simulink model "simulink_mecha"  (R2016b)
settings: Solver=VariableStepAuto  StartTime=0.0  StopTime=50  RelTol=1e-3
libraries: aerolibutil x1, simulink x1
settings Model: Creator=Utente  LastModifiedBy=Utente

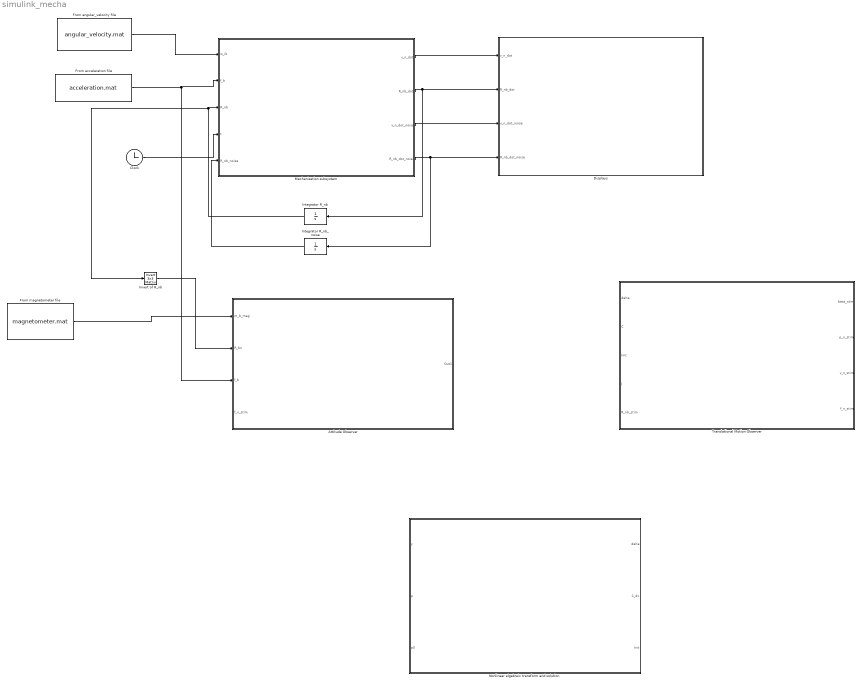
== system simulink_mecha ==
  Attitude Observer : Subsystem
  Clock : Clock
  Displays : Subsystem
  From acceleration file : FromFile  FileName=acceleration.mat  SampleTime=0
  From angular_velocity file : FromFile  FileName=angular_velocity.mat  SampleTime=0
  From magnetometer file : FromFile  FileName=magnetometer.mat  SampleTime=0  InterpolationWithinTimeRange=Zero order hold
  Integrator R_nb : Integrator
  Integrator R_nb_noise : Integrator
  Invert of R_nb : aerolibutil/Invert  3x3 Matrix
  Mechanisation subsystem : Subsystem
  Nonlinear algebraic transform and solution : Subsystem
  Translational Motion Observer : Subsystem
  wires:
  From angular_velocity file/1 -> Mechanisation subsystem/1(w_ib)
  From acceleration file/1 -> Mechanisation subsystem/2(f_b), Attitude Observer/3(f_b)
  Clock/1 -> Mechanisation subsystem/4(t)
  Mechanisation subsystem/2(R_nb_dot) -> Integrator R_nb/1, Displays/2(R_nb_dot)
  Integrator R_nb/1 -> Invert of R_nb/1, Mechanisation subsystem/3(R_nb)
  Mechanisation subsystem/1(v_n_dot) -> Displays/1(v_n_dot)
  Mechanisation subsystem/3(v_n_dot_noise) -> Displays/3(v_n_dot_noise)
  Mechanisation subsystem/4(R_nb_dot_noise) -> Integrator R_nb_noise/1, Displays/4(R_nb_dot_noise)
  Integrator R_nb_noise/1 -> Mechanisation subsystem/5(R_nb_noise)
  Invert of R_nb/1 -> Attitude Observer/2(R_bn)
  From magnetometer file/1 -> Attitude Observer/1(m_b_mag)

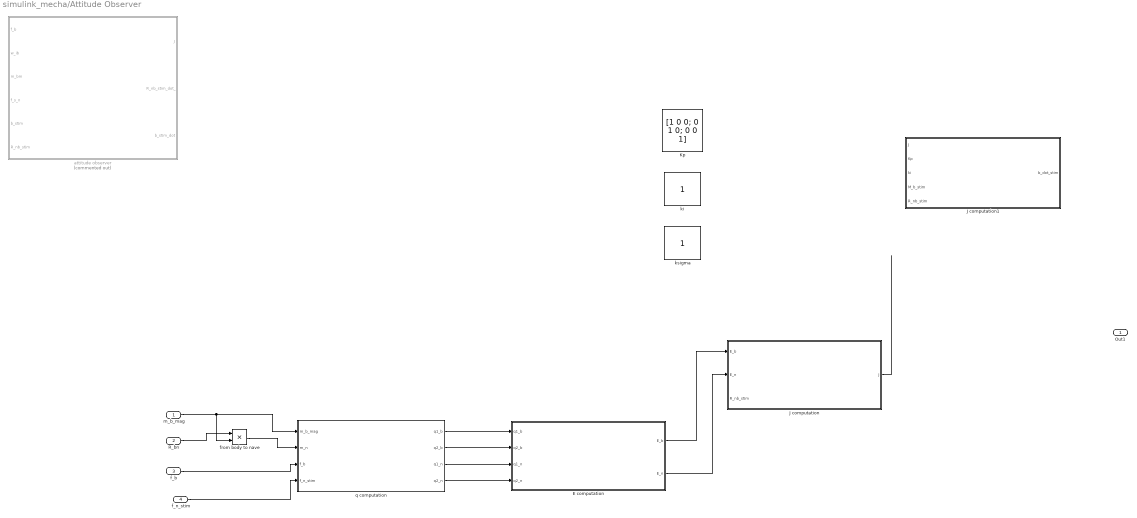
== system simulink_mecha/Attitude Observer ==
  m_b_mag : Inport
  R_bn : Inport  Port=2
  f_b : Inport  Port=3
  f_n_stim : Inport  Port=4
  E computation : MATLAB Function  TreatAsAtomicUnit=on
  J computation : MATLAB Function  TreatAsAtomicUnit=on
  J computation1 : MATLAB Function  TreatAsAtomicUnit=on
  Kp : Constant  Value=[1 0 0; 0 1 0; 0 0 1]
  attitude observer : MATLAB Function  Commented=on  TreatAsAtomicUnit=on
  from body to nave : Product
  ki : Constant
  ksigma : Constant
  q computation : MATLAB Function  TreatAsAtomicUnit=on
  Out1 : Outport
  wires:
  m_b_mag/1 -> from body to nave/2, q computation/1(m_b_mag)
  R_bn/1 -> from body to nave/1
  f_b/1 -> q computation/3(f_b)
  f_n_stim/1 -> q computation/4(f_n_stim)
  from body to nave/1 -> q computation/2(m_n)
  q computation/1(q1_b) -> E computation/1(q1_b)
  q computation/2(q2_b) -> E computation/2(q2_b)
  q computation/3(q1_n) -> E computation/3(q1_n)
  q computation/4(q2_n) -> E computation/4(q2_n)
  E computation/1(E_b) -> J computation/1(E_b)
  E computation/2(E_n) -> J computation/2(E_n)
  ? -> J computation/3(R_nb_stim)
  J computation/1(J) -> ?

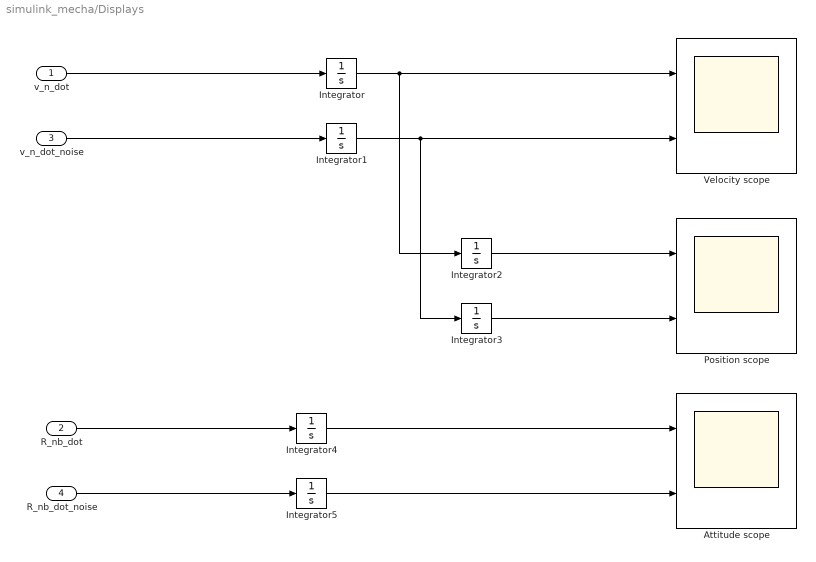
== system simulink_mecha/Displays ==
  v_n_dot : Inport
  R_nb_dot : Inport  Port=2
  v_n_dot_noise : Inport  Port=3
  R_nb_dot_noise : Inport  Port=4
  Attitude scope : Scope  NumInputPorts=2
  Integrator{,1..5} (6 alike) : Integrator
  Position scope : Scope  NumInputPorts=2
  Velocity scope : Scope  NumInputPorts=2
  wires:
  v_n_dot/1 -> Integrator/1
  v_n_dot_noise/1 -> Integrator1/1
  Integrator/1 -> Integrator2/1, Velocity scope/1
  Integrator1/1 -> Integrator3/1, Velocity scope/2
  Integrator2/1 -> Position scope/1
  Integrator3/1 -> Position scope/2
  R_nb_dot/1 -> Integrator4/1
  R_nb_dot_noise/1 -> Integrator5/1
  Integrator4/1 -> Attitude scope/1
  Integrator5/1 -> Attitude scope/2

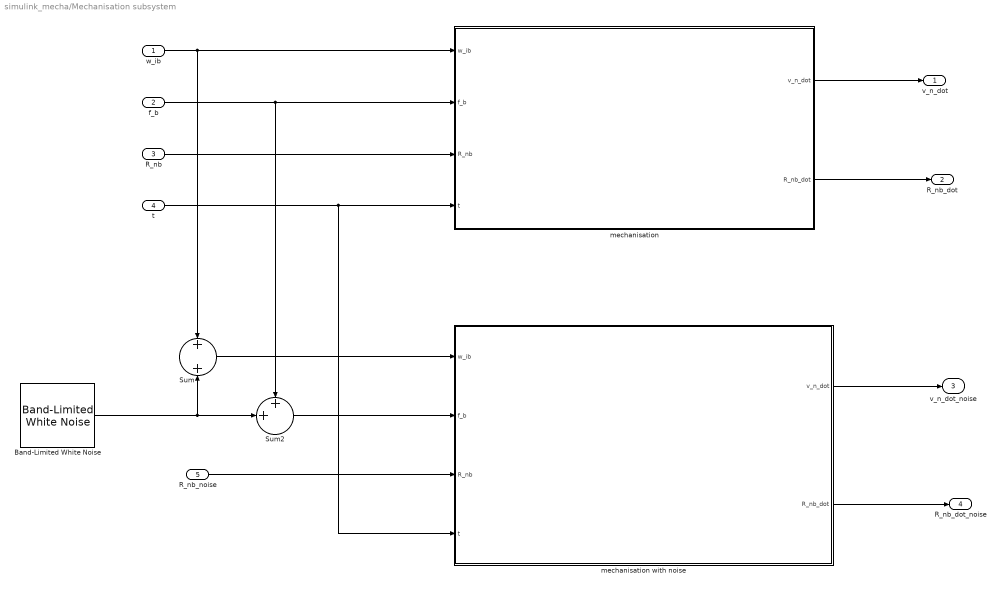
== system simulink_mecha/Mechanisation subsystem ==
  w_ib : Inport
  f_b : Inport  Port=2
  R_nb : Inport  Port=3
  t : Inport  Port=4
  R_nb_noise : Inport  Port=5
  Band-Limited White Noise : simulink/Sources/Band-Limited White Noise  Cov=[100 100 100]'  Ts=0.1  seed=[23341]  VectorParams1D=off
  Sum : Sum  Inputs=+|+
  Sum2 : Sum  Inputs=++|
  mechanisation : MATLAB Function  TreatAsAtomicUnit=on
  mechanisation with noise : MATLAB Function  TreatAsAtomicUnit=on
  v_n_dot : Outport
  R_nb_dot : Outport  Port=2
  v_n_dot_noise : Outport  Port=3
  R_nb_dot_noise : Outport  Port=4
  wires:
  w_ib/1 -> mechanisation/1(w_ib), Sum/1
  t/1 -> mechanisation with noise/4(t), mechanisation/4(t)
  R_nb/1 -> mechanisation/3(R_nb)
  f_b/1 -> Sum2/1, mechanisation/2(f_b)
  mechanisation/1(v_n_dot) -> v_n_dot/1
  mechanisation/2(R_nb_dot) -> R_nb_dot/1
  Band-Limited White Noise/1 -> Sum/2, Sum2/2
  Sum/1 -> mechanisation with noise/1(w_ib)
  Sum2/1 -> mechanisation with noise/2(f_b)
  mechanisation with noise/1(v_n_dot) -> v_n_dot_noise/1
  mechanisation with noise/2(R_nb_dot) -> R_nb_dot_noise/1
  R_nb_noise/1 -> mechanisation with noise/3(R_nb)

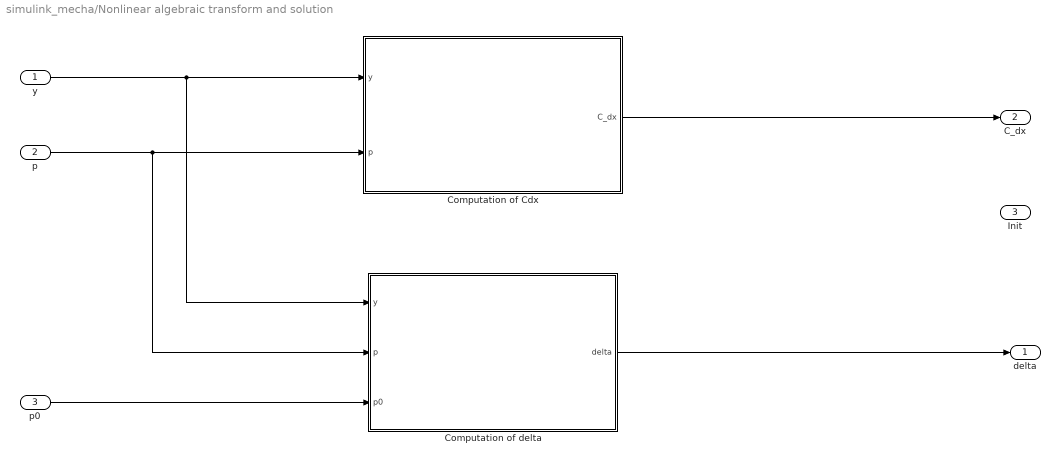
== system simulink_mecha/Nonlinear algebraic transform and solution ==
  y : Inport
  p : Inport  Port=2
  p0 : Inport  Port=3
  Computation of Cdx : MATLAB Function  TreatAsAtomicUnit=on
  Computation of delta : MATLAB Function  TreatAsAtomicUnit=on
  delta : Outport
  C_dx : Outport  Port=2
  Init : Outport  Port=3
  wires:
  y/1 -> Computation of delta/1(y), Computation of Cdx/1(y)
  p/1 -> Computation of delta/2(p), Computation of Cdx/2(p)
  p0/1 -> Computation of delta/3(p0)
  Computation of Cdx/1(C_dx) -> C_dx/1
  Computation of delta/1(delta) -> delta/1

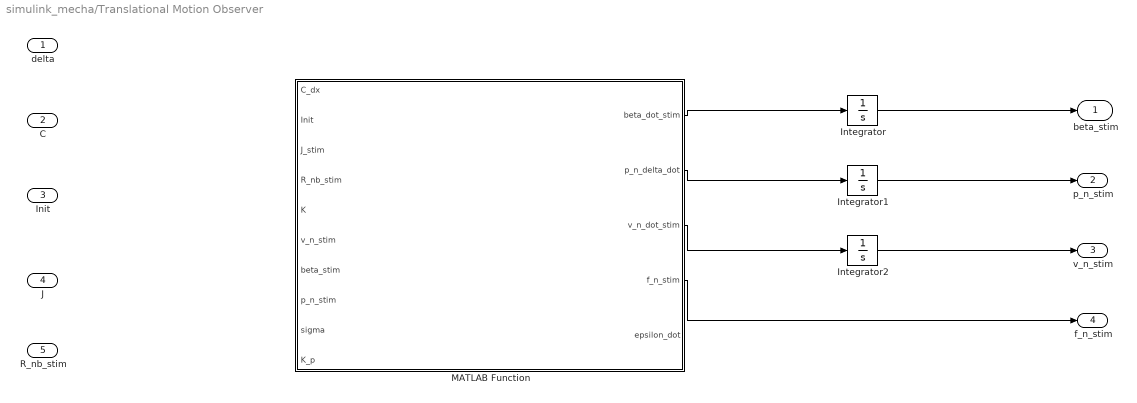
== system simulink_mecha/Translational Motion Observer ==
  delta : Inport
  C : Inport  Port=2
  Init : Inport  Port=3
  J : Inport  Port=4
  R_nb_stim : Inport  Port=5
  Integrator : Integrator
  Integrator1 : Integrator
  Integrator2 : Integrator
  MATLAB Function : MATLAB Function  TreatAsAtomicUnit=on
  beta_stim : Outport
  p_n_stim : Outport  Port=2
  v_n_stim : Outport  Port=3
  f_n_stim : Outport  Port=4
  wires:
  MATLAB Function/4(f_n_stim) -> f_n_stim/1
  MATLAB Function/3(v_n_dot_stim) -> Integrator2/1
  Integrator2/1 -> v_n_stim/1
  MATLAB Function/2(p_n_delta_dot) -> Integrator1/1
  Integrator1/1 -> p_n_stim/1
  Integrator/1 -> beta_stim/1
  MATLAB Function/1(beta_dot_stim) -> Integrator/1

== matlab function simulink_mecha/Attitude Observer/E computation ==
  data: q1_b input; E_b output; q2_b input; q1_n input; q2_n input; E_n output
function [E_b, E_n]= Efunc(q1_b, q2_b, q1_n, q2_n)



E_b = (q1_b, skew(q1_b)*q2_b, (skew(q1_b)*skew(q1_b))*q2_b);
E_n = (q1_n, skew(q1_n)*q2_n, (skew(q1_n)*skew(q1_n))*q2_n);

== matlab function simulink_mecha/Attitude Observer/q computation ==
  data: m_b_mag input; q1_b output; m_n input; f_b input; f_n_stim input; q2_b output; q1_n output; q2_n output
function [q1_b, q2_b, q1_n, q2_n] = qfunc(m_b_mag, m_n, f_b, f_n_stim)

g_n = [0 0 1]';

q1_b = m_b_mag/norm(m_b_mag,2);
q2_b = f_b/norm(g_n,2);

q1_n = m_n/norm(m_n,2);
q2_n = f_n_stim/norm(g_n,2);

== matlab function simulink_mecha/Attitude Observer/attitude observer ==
  data: f_b input; J output; w_ib input; m_bm input; f_s_n input; b_stim input; R_nb_stim input; R_nb_stim_dot_ output; b_stim_dot output
function [J, R_nb_stim_dot_, b_stim_dot] = fcn(f_b, w_ib, m_bm, f_s_n, b_stim, R_nb_stim)

g_n = [0 0 1];

Skew = zeros(3,3);
Skew(1,2) = -(w_ib(3) - b_stim(3));
Skew(2,1) = (w_ib(3) - b_stim(3));
Skew(1,3) = (w_ib(2) - b_stim(2));
Skew(3,1) = -(w_ib(2) - b_stim(2));
Skew(2,3) = -(w_ib(1) - b_stim(1));
Skew(3,2) = (w_ib(1) - b_stim(1));

Kp = eye(3); % gain matrix
sigma = 1; % sigma >= 1

J_func = eye(3);
R_nb_stim_dot = R_nb_stm * Skew + sigma * Kp * J_func;

% b_stim_dot = Proj

q1_b = m_bmag/norm(m_bmag,2);
q2_b = f_b/norm(g_n,2);

q1_n = m_n/norm(m_n,2);
q2_n = f_s_n/norm(g_n,2);



E_b = (q1_b, Skew(q1_b)*q2_b, (S(q1_b)*S(q1_b))*q2_b);
E_n = (q1_n, Skew(q1_n)*q2_n, (S(q1_n)*S(q1_n))*q2_n);

J = (E_n - R_nb_stim * E_b) * (E_b');

== matlab function simulink_mecha/Mechanisation subsystem/mechanisation ==
  data: w_ib input; f_b input; v_n_dot output; R_nb_dot output; R_nb input; t input
function [v_n_dot, R_nb_dot] = mechanisation(w_ib, f_b, R_nb, t)



g_n = [0 0 1]';

% w_ib = size(3,1);

if t == 0
    v_n_dot = zeros(3,1);
    R_nb_dot = zeros(3,3);
    R_nb = eye(3);
end

% mechanisation

% Skew = zeros(3,3);
% Skew(1,2) = -w_ib(3);
% Skew(2,1) = w_ib(3);
% Skew(1,3) = w_ib(2);
% Skew(3,1) = -w_ib(2);
% Skew(2,3) = -w_ib(1);
% Skew(3,2) = w_ib(1);

Skew = skew(w_ib);


%p_dot = v_n;
v_n_dot = R_nb * f_b + g_n;
R_nb_dot = R_nb * Skew;

== matlab function simulink_mecha/Mechanisation subsystem/mechanisation with noise ==
  data: w_ib input; f_b input; v_n_dot output; R_nb_dot output; R_nb input; t input
function [v_n_dot, R_nb_dot] = mechanisation(w_ib, f_b, R_nb, t)



g_n = [0 0 1]';

% w_ib = size(3,1);

if t == 0
    v_n_dot = zeros(3,1);
    R_nb_dot = zeros(3,3);
    R_nb = eye(3);
end

% mechanisation

% Skew = zeros(3,3);
% Skew(1,2) = -w_ib(3);
% Skew(2,1) = w_ib(3);
% Skew(1,3) = w_ib(2);
% Skew(3,1) = -w_ib(2);
% Skew(2,3) = -w_ib(1);
% Skew(3,2) = w_ib(1);
Skew = skew(w_ib);


%p_dot = v_n;
v_n_dot = R_nb * f_b + g_n;
R_nb_dot = R_nb * Skew;

== matlab function simulink_mecha/Attitude Observer/J computation ==
  data: E_b input; J output; E_n input; R_nb_stim input
function J = Jfunc(E_b, E_n, R_nb_stim)


J = (E_n - R_nb_stim * E_b) * (E_b');

== matlab function simulink_mecha/Attitude Observer/J computation1 ==
  data: J input; b_dot_stim output; Kp input; ki input; M_b_stim input; R_nb_stim input
function b_dot_stim = b_dot_stim_func(J, Kp, ki, M_b_stim, R_nb_stim)

% function Pa(A)

== matlab function simulink_mecha/Translational Motion Observer/MATLAB Function ==
  data: C_dx input; beta_dot_stim output; Init input; J_stim input; R_nb_stim input; p_n_delta_dot output; v_n_dot_stim output; f_n_stim output; K input; v_n_stim input; beta_stim input; p_n_stim input; sigma input; K_p input; epsilon_dot output
function [beta_dot_stim,p_n_delta_dot,v_n_dot_stim,f_n_stim,epsilon_dot] =  tmo_func(C_dx,Init,J_stim,R_nb_stim, K, v_n_stim, beta_stim, p_n_stim,sigma,K_p)

% K = [K_pp; K_beta_p; K_v_p; K_eps_p] obtained by Riccati equation..
% damn..

% remember to insert a clock to define dimensions of all variables

g_n = [0 0 1]';

x_stim = [p_n_deta beta_stim];
delta_stim = 2*C_dx*x_stim;
delta_ = (delta - delta_stim);



p_n_delta_dot = v_n_stim + K_pp * delta_;        % eq 14


beta_dot_stim = K_beta_p * delta_;                       % eq 15


%theoretically we can't know epsilon
f_n_stim = R_nb_stim*f_b_imu + epsilon ;         % eq 18


v_n_dot_stim  = f_n_stim + g_n + K_v_p*delta_;         % eq 16


epsilon_dot   = -sigma*K_p*J_stim*f_b_imu + K_eps_p*delta_; % eq 17
end

== matlab function simulink_mecha/Nonlinear algebraic transform and solution/Computation of Cdx ==
  data: y input; C_dx output; p input
function C_dx  = C_dx_func(y,p)

    % y vector 
    % p matrix has row vectors
    %            (x,y,z) cols 
    %            m-rows are the numbers of the transponders
    % all variables are in navigation frame oh yeah! baby ;)
    
    [row,col] = size(p);
    [row_,col_] = size(y);
    
    % m-measure vector
    p_m = p(row);
    y_m = y(row);

    
    p_ = [];
    y_ = [];
    
    for i = 1 : 1 : row-1
    
        p_ = [p_ ; p_m - p(i,:)];
        y_ = [y_ ; y(i) - y_m];
        
    end
    
    C_dx = [p_ y_];

end

== matlab function simulink_mecha/Nonlinear algebraic transform and solution/Computation of delta ==
  data: y input; delta output; p input; p0 input
function delta  = delta_func(y,p,p0)

    % y vector 
    % p matrix has row vectors
    %            (x,y,z) cols 
    %            m-rows are the numbers of the transponders
    % all variables are in navigation frame oh yeah! baby ;)
    % z is a col vector of scalars
    
    [row,col] = size(p);
    [row_,col_] = size(y);
    
   
    %defining los vector
    
    for i = 1:1:row
        
       p_los(i,:) = p(i,:) - p0;
       z(i) = y(i)^2 - norm(p_los(i,:))^2;
        
    end    
    
    for i = 1:1:row-1
       
        delta(i) = z(i) - z_m ; %amm fenito
        
    end

end
